simulink model "holidays9"  (R2019a)
settings: Solver=VariableStepAuto  StartTime=0.0  StopTime=10.0  RelTol=1e-3
settings Model: Creator=Aditya  LastModifiedBy=Aditya

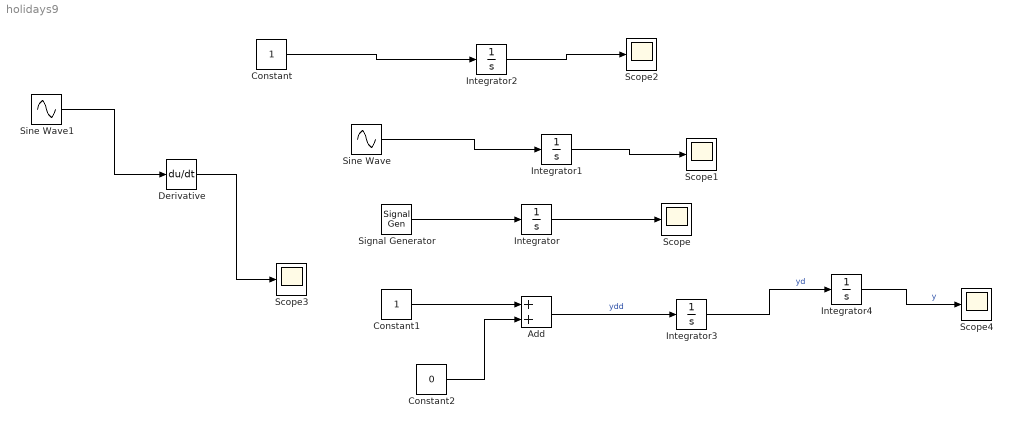
== system holidays9 ==
  Add : Sum
  Constant : Constant
  Constant1 : Constant
  Constant2 : Constant  Value=0
  Derivative : Derivative
  Integrator{,1..4} (5 alike) : Integrator
  Scope{,1..4} (5 alike) : Scope
  Signal Generator : SignalGenerator  WaveForm=square  Units=rad/sec
  Sine Wave : Sin  SampleTime=0
  Sine Wave1 : Sin  SampleTime=0
  wires:
  Signal Generator/1 -> Integrator/1
  Integrator/1 -> Scope/1
  Sine Wave/1 -> Integrator1/1
  Integrator1/1 -> Scope1/1
  Constant/1 -> Integrator2/1
  Integrator2/1 -> Scope2/1
  Sine Wave1/1 -> Derivative/1
  Derivative/1 -> Scope3/1
  Constant1/1 -> Add/1
  Add/1 -> Integrator3/1  "ydd"
  Integrator3/1 -> Integrator4/1  "yd"
  Integrator4/1 -> Scope4/1  "y"
  Constant2/1 -> Add/2
